simulink model "untitled"  (R2022a)
settings: Solver=VariableStepAuto  StartTime=0.0  StopTime=1  RelTol=1e-3
libraries: cstblocks x1
settings Model: Creator=hardi  LastModifiedBy=hardi

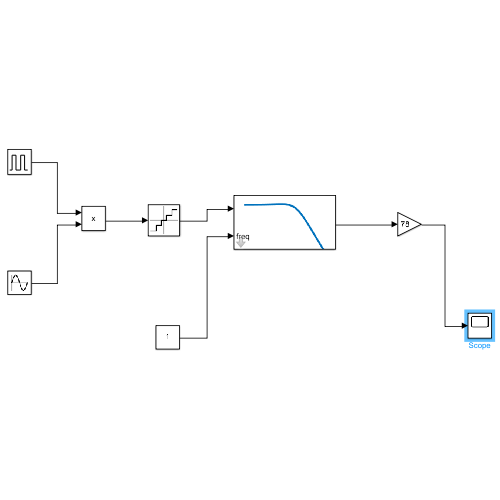
[thumbnail: Simulink's stored preview of the top-level diagram]
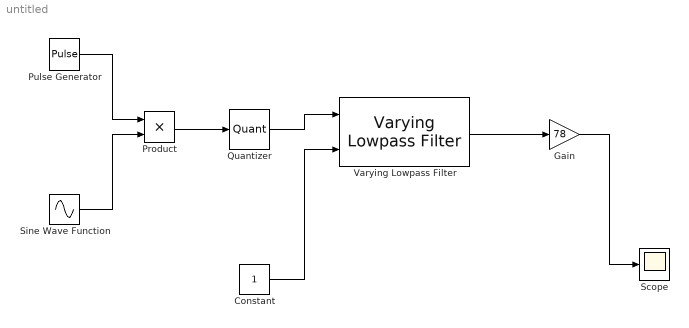
== system untitled ==
  Constant : Constant
  Gain : Gain  Gain=78
  Product : Product
  Pulse Generator : DiscretePulseGenerator  PulseType=Time based  Amplitude=5  Period=0.02/32  PulseWidth=50
  Quantizer : Quantizer  QuantizationInterval=0.1  LinearizeAsGain=off
  Scope : Scope
  Sine Wave Function : Sin  Frequency=2^pi*50  SampleTime=0
  Varying Lowpass Filter : cstblocks/Linear Parameter Varying/Varying Lowpass Filter  N=1
  wires:
  Sine Wave Function/1 -> Product/2
  Pulse Generator/1 -> Product/1
  Product/1 -> Quantizer/1
  Quantizer/1 -> Varying Lowpass Filter/1
  Constant/1 -> Varying Lowpass Filter/2
  Varying Lowpass Filter/1 -> Gain/1
  Gain/1 -> Scope/1
